simulink model "flightControlSystem"  (R2024b)
settings: Solver=ode3  StartTime=0  StopTime=TFinal  FixedStep=Ts  RelTol=1e-3  EnableMultiTasking=on
model workspace (MAT data in the model file):
  CIRCLE_PTS = [19 19 19]
  ZEROS = [0 0 0 0 0 0 0 0 0 0 0 0 ... (1444 elements, 38x38)]
undefined symbols (not defined in the file or in its folder): codertarget, Controller, DiscIntNeverNeededParam, Discrete, Estimator, g, gray, init, Sensors, Time, Ts, var_acc_angle_N, var_bias_gyr_N, var_gyro_p_N, Vehicle
libraries: simulink x37, slpidlib x4, ctrlSharedLib x4, sharedtransform x3, visiontextngfix x1, parrotlib x1
(part 3 of 3)

== matlab function flightControlSystem/Image Processing System/check_previous_target ==
  data: bw_image input; is_scan output; in_red output; prev_xy input; DISTANCE input; target output; compare output
function [is_scan, in_red, target,compare]  = fcn(bw_image, prev_xy, DISTANCE)

prev_x = prev_xy(1);
prev_y = prev_xy(2);

in_red = bw_image(60, 80);
compare = ~in_red;

is_scan = 0;
target_x = 1;
target_y = 1;
speed = 0;

if prev_x == 0 || prev_y == 0 %scan when prev_coordinates unvalid
    is_scan = 1;
else 
    if bw_image(prev_x, prev_y) == 1 %prev_coordinates in red

        %continue upload new coordinats
        [ref_x, ref_y] = middle_point_of_endless_line(bw_image, prev_x, prev_y);

        target_x = prev_x + ref_x;
        target_y = prev_y + ref_y;
        
        %boundary limit. make path in image
        if target_y > 160
            if target_x == 120 
                target_x = 120 - mod(target_y, 160);
            elseif target_x == 1 
                target_x = mod(target_y, 160);
            end
            target_y = 160;
            
        elseif target_y < 1
            if target_x == 120 
                target_x = 120 - abs(target_y);
            elseif target_x == 1 
                target_x = abs(target_y); 
            end
            target_y = 1;
            
        elseif target_x < 1
            if target_y == 160
                target_y = 160 - abs(target_x);
            elseif target_y == 1
                target_y = abs(target_x);
            end
            target_x = 1;
            
        elseif target_x > 120
            if target_y == 160
                target_y = 160 - (target_x - 120);
            elseif target_y == 1
                target_y = target_x - 120;
            end
            target_x = 120;
        end

        %{
        if target_x < 1   target_x = 1;   end
        if target_x > 120 target_x = 120; end
        if target_y < 1   target_y = 1;   end
        if target_y > 160 target_y = 160; end
        %}
        speed = 100;

    else %target not in red
        
        % endless dissappeared ----------------------------
        if in_red
            distance = line_drawer(60, 80, prev_x, prev_y, bw_image, compare);
            if distance < DISTANCE
                is_scan = 1;
                speed = 0;
            else
                speed = distance;
            end
            
            target_x = prev_x;
            target_y = prev_y;
        else
            is_scan = 1;
            target_x = prev_x;
            target_y = prev_y;
            speed = 40;
        end

    end
end
target = [target_x, target_y, speed];

end % func end



function [ref_x, ref_y] = middle_point_of_endless_line(bw_image, target_x, target_y)

w = edge_number(target_x, target_y);

if w == 1 || w == 3

    % to right
    iter_y = target_y;
    iter_x = target_x;
    plus_or_minus = 1;
    x_or_y = 0; % 0:y   1:x
    distance = 0;

    while bw_image(iter_x, iter_y) == 1
        if x_or_y == 0
            iter_y = iter_y + plus_or_minus;
        else
            iter_x = iter_x + plus_or_minus;
        end
        distance = distance + 1;
        
        if iter_y > 160
            iter_y = 160;
            x_or_y = 1;
            if iter_x == 120
                plus_or_minus = -1;
            elseif iter_x == 1
                plus_or_minus = 1;
            end
        end
        if iter_x < 1
            break;
        elseif iter_x > 120
            break;
        end
    end
    right = distance;

    % to left
    iter_y = target_y;
    iter_x = target_x;
    plus_or_minus = -1;
    x_or_y = 0; % 0:y   1:x
    distance = 0;
    
    while bw_image(iter_x, iter_y) == 1
        if x_or_y == 0
            iter_y = iter_y + plus_or_minus;
        else
            iter_x = iter_x + plus_or_minus;
        end
        distance = distance + 1;

        if iter_y < 1
            iter_y = 1;
            x_or_y = 1;
            if iter_x == 120
                plus_or_minus = -1;
            elseif iter_x == 1
                plus_or_minus = 1;
            end
        end
        if iter_x < 1
            break
        elseif iter_x > 120
            break
        end
    end
    left = distance;
    
    
    ref_x = 0;
    diff = right - left;
    
    if abs(diff) >= 7 && abs(diff) < 25
        ref_y = round(diff/2);
    else
        ref_y = 0;
    end

else % ------------------------- 2 & 4 --------------------------
    % to up
    iter_x = target_x;
    iter_y = target_y;
    plus_or_minus = -1;
    x_or_y = 1; % 0:y   1:x
    distance = 0;
    while bw_image(iter_x, iter_y) == 1
        if x_or_y == 0
            iter_y = iter_y + plus_or_minus;
        else
            iter_x = iter_x + plus_or_minus;
        end
        distance = distance + 1;

        if iter_x < 1
            iter_x = 1;
            x_or_y = 0;
            if iter_y == 1
                plus_or_minus = 1;
            elseif iter_y == 160
                plus_or_minus = -1;
            end
        end
        if iter_y > 160
            break
        elseif iter_y < 1
            break
        end
    end
    up = distance;

    % to down
    iter_x = target_x;
    iter_y = target_y;
    plus_or_minus = 1;
    x_or_y = 1; % 0:y   1:x
    distance = 0;
    while bw_image(iter_x, iter_y) == 1
        if x_or_y == 0
            iter_y = iter_y + plus_or_minus;
        else
            iter_x = iter_x + plus_or_minus;
        end
        distance = distance + 1;
        if iter_x > 120
            x_or_y = 0;
            iter_x = 120;
            if iter_y == 1
                plus_or_minus = 1;
            elseif iter_y == 160
                plus_or_minus = -1;
            end
        end
        if iter_y > 160
            break;
        elseif iter_y < 1
            break;
        end
    end
    down = distance;

    diff = down - up;

    ref_y = 0;
    if abs(diff) >= 7 && abs(diff) < 25
        ref_x = round(diff/2);
    else
        ref_x = 0;
    end
end

end

== matlab function flightControlSystem/Image Processing System/circle_detection_landing ==
  data: bw_image input; detected output; way output; shape input
function [detected, way] = fcn(bw_image, shape)

persistent landing;
if isempty(landing)
    landing = 0;
end

detected = 0;
way = [0 0 0];
land = 0;

%landing order
if landing == 1
    way = [0 0 1];
    detected = 1;

else
    [total_pixel, cord_x, cord_y] = detect_circle(bw_image, shape);
    
    if total_pixel >= 1350%circle detection parameters
        detected = 1;
        center_x = cord_x + 19;%shape parameters
        center_y = cord_y + 19;%shape parameters
    
        %Image boundary limit
        if center_x > 120
            center_x = 120;
        end
        if center_y > 160
            center_y = 160;
        end
        
        %landing order limit
        dif_x = round(60 - center_x);
        dif_y = round(center_y - 80);
        %calculate 
        dist = sqrt(dif_x * dif_x + dif_y * dif_y);
    
        fprintf(' #### CIRCLE - centers: %3.1f %3.1f | dist: %3.1f\n', ...
            center_x, center_y, dist);
    
        if dist < 15
            land = 1;
            landing = 1;
        end
        way_x = dif_x / 130000;
        way_y = dif_y / 130000;
        way = [way_x way_y land];
    end

end

end

function [total_pixel, cord_x, cord_y] = detect_circle(bw_image, shape)

%  total_pixel: sum of number of pixel
%       cord_x: row coordinate of bw_image
%       cord_y: column coordinate of bw_image

[circle_size_x, circle_size_y] = size(shape);
R = 120;  C = 160;

total_pixel = 0;
cord_x = 0;
cord_y = 0;

%circle detection, a slide window
for i = 1:(R - circle_size_x)
    for j = 1:(C - circle_size_y)
        section = bw_image(i:i+circle_size_x-1, j:j+circle_size_y-1);
        result = sum(~xor(section, shape), 'all');
        if result > total_pixel
            total_pixel = result;
            cord_x = i;
            cord_y = j;
        end
    end

end
end

== matlab function flightControlSystem/Image Processing System/visualize_helper ==
  data: r input; R output; g input; b input; way_x input; way_y input; G output; B output; lx input; ly input; rx input; ry input
function [R,G,B] = fcn(r,g,b, way_x, way_y,  lx,ly, rx,ry)

% completely unnecessary block for algorithm, just for visualize

r(60,80) = 255; g(60,80) = 255; b(60,80) = 255;

if way_x >= 1 && way_y >= 1 && way_x <= 120 && way_y <= 160


% -----------------------------------------------
    x1 = 60; y1 = 80;  x2 = way_x;   y2 = way_y;
    swapepd = 0;
    if abs(y2 - y1) > abs(x2 - x1)
        %disp('[swapped] dy bigger')
        swapepd = 1;
        [x1,y1] = deal(y1,x1);
        [x2,y2] = deal(y2,x2);
        xk = 1; yk = 1;
        if (x2 < x1) xk = -1; end
        if (y2 < y1) yk = -1; end
    else
        xk = -1; yk = -1;
        if (x2 > x1) xk = 1; end
        if (y2 > y1) yk = 1; end

    end
    dy = abs(y2-y1);
    dx = abs(x2-x1);
    % --------------------------------------
    m = 2 * dy;
    slope_error = m - 2*dx;
  
    y = y1;
    for x = x1:xk:x2
        if swapepd == 1
            r(y,x) = 255; g(y,x) = 255; b(y,x) = 255;
        else
            r(x,y) = 255; g(x,y) = 255; b(x,y) = 255;
        end
        
   
        slope_error = slope_error + m;
        if (slope_error > 0)
            y = y + yk;
            slope_error = slope_error - 2 * dx;
        end
    end
end




% --------------------------------------------
x1 = 60; y1 = 80; x2 = lx; y2 = ly;
    swapepd = 0;
    if abs(y2 - y1) > abs(x2 - x1)
        %disp('[swapped] dy bigger')
        swapepd = 1;
        [x1,y1] = deal(y1,x1);
        [x2,y2] = deal(y2,x2);
        xk = 1; yk = 1;
        if (x2 < x1) xk = -1; end
        if (y2 < y1) yk = -1; end
    else
        xk = -1; yk = -1;
        if (x2 > x1) xk = 1; end
        if (y2 > y1) yk = 1; end

    end
    dy = abs(y2-y1);
    dx = abs(x2-x1);
    % --------------------------------------
    m = 2 * dy;
    slope_error = m - 2*dx;
  
    y = y1;
    for x = x1:xk:x2
        if swapepd == 1
            g(y,x) = 255;
        else
            g(x,y) = 255;
        end
        
   
        slope_error = slope_error + m;
        if (slope_error > 0)
            y = y + yk;
            slope_error = slope_error - 2 * dx;
        end
    end
% -----------------------------------------

    x1 = 60; y1 = 80; x2 = rx; y2 = ry;
    swapepd = 0;
    if abs(y2 - y1) >= abs(x2 - x1)
        %disp('[swapped] dy bigger')
        swapepd = 1;
        [x1,y1] = deal(y1,x1);
        [x2,y2] = deal(y2,x2);
        xk = 1; yk = 1;
        if (x2 < x1) xk = -1; end
        if (y2 < y1) yk = -1; end
    else
        xk = -1; yk = -1;
        if (x2 > x1) xk = 1; end
        if (y2 > y1) yk = 1; end

    end
    dy = abs(y2-y1);
    dx = abs(x2-x1);
    % --------------------------------------
    m = 2 * dy;
    slope_error = m - 2*dx;
  
    y = y1;
    for x = x1:xk:x2
        if swapepd == 1
            if x <1 break; end
            g(y,x) = 255;
        else
            g(x,y) = 255;
        end
        
   
        slope_error = slope_error + m;
        if (slope_error > 0)
            y = y + yk;
            slope_error = slope_error - 2 * dx;
        end
    end

b(40:80, 60:90) = 200;
R = r;
G = g;
B = b;
end

== matlab function flightControlSystem/Image Processing System/write_or_not ==
  data: target input; way_out output; in_red input; prev_xy input; target_x output; target_y output
function [way_out, target_x, target_y] = fcn(target, in_red, prev_xy)

x = target(1);
y = target(2);
speed = target(3);

if in_red
    X = x;   Y = y;
    target_x = x;  target_y = y;%output as a valid target
else
    X = x;  Y = y; 
    target_x = prev_xy(1);  
    target_y = prev_xy(2);%dont move and start a new loop
end

way_out = [X Y speed];

%fprintf('X = %f | Y = %f\n', target_x, target_y);
end

== matlab function flightControlSystem/Image Processing System/MATLAB Function ==
  data: rgb_image input; bw_image output
function bw_image = red_detection_binarize(rgb_image)
    %  RGB To HSV
    hsv_image = rgb2hsv(rgb_image);

    % HSV Parameters_red
    h_min = 0;    % Min Hue 
    h_max = 0.1;  % Max Hue
    s_min = 0.3;  % Min Saturation
    s_max = 1;    % Max Saturation
    v_min = 0.1;  % Min Value
    v_max = 1;    % Max Value

    % Mask 
    mask1 = (hsv_image(:,:,1) >= h_min & hsv_image(:,:,1) <= h_max) & ...
            (hsv_image(:,:,2) >= s_min & hsv_image(:,:,2) <= s_max) & ...
            (hsv_image(:,:,3) >= v_min & hsv_image(:,:,3) <= v_max);
    mask2 = (hsv_image(:,:,1) >= 0.9 & hsv_image(:,:,1) <= 1) & ...
            (hsv_image(:,:,2) >= s_min & hsv_image(:,:,2) <= s_max) & ...
            (hsv_image(:,:,3) >= v_min & hsv_image(:,:,3) <= v_max);

    % Mask Sum
    red_mask = mask1 | mask2;

    % Keep red  mask, set others black
    masked_rgb = rgb_image;
    masked_rgb(repmat(~red_mask, [1, 1, 3])) = 0;

    % Mask To Grey
    gray_image = rgb2gray(masked_rgb);

    % Grey To Binizaration
    level = graythresh(gray_image);       % Calculate threshold
    bw_image = imbinarize(gray_image, level); 

    % Noise Filter
    %u = bwareaopen(u, 50);
end

== matlab function flightControlSystem/Control System/Controller/Position Controller/Position error transformation (Earth to Body frame) ==
  data: yaw input; xy_err_earth input; xy_err_body output
function xy_err_body = fcn(yaw,xy_err_earth)

transformation = [cos(yaw), sin(yaw); -sin(yaw),  cos(yaw)];
xy_err_body = transformation * xy_err_earth;


end

== matlab function flightControlSystem/Image Processing System/speed_calculator ==
  data: target input; X output; Y output
function [X,Y] = fcn(target)

x = target(1);
y = target(2);
speed = target(3);

if speed == 100
    speed = 200;
elseif speed < 60
    speed = 60;
end


X = (60-x) / 10000000 * speed;
Y = (y-80) / 10000000 * speed;


%fprintf(' --- speed: %f | ', speed); fprintf('vectors: X=%.5f | Y=%.5f\n', X, Y);

end

== matlab function flightControlSystem/Image Processing System/Feedback Control ==
  data: target_x output; prev_xy input; target_y output
function [target_x, target_y] = fcn(prev_xy)

    x = prev_xy(1);
    y = prev_xy(2);
    
    if x == 0 || y == 0 %initial satate
        target_x = 0;
        target_y = 0;
    else
        target_x = 60 + (60 - x) + 1; %1--120
        target_y = 80 + (80 - y) + 1; %2--159
    end

    %fprintf('opposite: %.0f %.0f -> %.0f %.0f\n', x, y, way_x, way_y);
end

== matlab function flightControlSystem/Image Processing System/Position Corrector/center_vector_x ==
  data: bw_image input; slide_x output
function slide_x = fcn(bw_image) 
%input:bw_image,bw_image
%output:slide_x,x direction velocity

%initialize centerpoint
c1 = 60; 
c2 = 80;
left_p = 0;
right_p = 0;
center = bw_image(c1, c2);
compare = ~center;

%find left bound
for i = c2:-1:60 % <---  look left
    if bw_image(c1, i) == compare
        left_p = i;
        break
    end
end

%find right bound
for i = c2:100 % --->   look right
    if bw_image(c1, i) == compare
        right_p = i;
        break
    end
end

slide_x = 0;
if left_p ~= 0 && right_p ~= 0 % in line
    if center == 1
        vr = right_p - c2;  % length right 
        vl = c2 - left_p;   % length left
        diff = vr-vl;%calculate diff to center
        slide_x = get_speed(diff) * 20;%back to center
    end
end
end

function T = get_speed(t)

if t > 0 %too left
    if t < 1 %slowly adjust position when diif is small
        T = 0.000001;
    elseif t < 5
        T = 0.000002;
    elseif t < 10
        T = 0.000003;
    elseif t < 15
        T = 0.000004;
    elseif t < 20
        T = 0.000005;
    else
        T = 0.000006;
    end
else %too right
    if t < -20
        T = -0.000006;
    elseif t < -15
        T = -0.000005;
    elseif t < -10
        T = -0.000004;
    elseif t < -5
        T = -0.000003;
    elseif t < -1
        T = -0.000002;
    else
        T = -0.000001;
    end
end

end

== matlab function flightControlSystem/Image Processing System/range_points ==
  data: x input; x1 output; y input; ref input; y1 output; x2 output; y2 output
function [x1,y1, x2,y2] = get_range_points(x,y, ref)

% x1, y1 are left
% x2, y2 are right 
% according to center-to-edge vector.

W = edge_number(x,y);

if W == 1%up bound
    y1 = y - ref;%To left
    if y1 < 1
        x1 = x - y1;%become left
        y1 = 1;
    else
        x1 = x;
    end

    y2 = y + ref;%To right
    if y2 > 160
        x2 = y2-160;%become right
        y2 = 160;
    else
        x2 = x;
    end
elseif W == 2%left bound
    x1 = x + ref;
    if x1 > 120
        y1 = x1 - 120;
        x1 = 120;
    else
        y1 = y;
    end

    x2 = x - ref;
    if x2 < 1
        y2 = abs(x2) + 1;
        x2 = 1;
    else
        y2 = y;
    end
elseif W == 4%right bound
    x1 = x - ref;
    if x1 < 1
        y1 = 160 + x1;
        x1 = 1;
    else
        y1 = 160;
    end

    x2 = x + ref;
    if x2 > 120
        y2 = 160 - (x2 - 120);
        x2 = 120;
    else
        y2 = y;
    end
elseif W == 3%down bound
    y1 = y + ref;%159+70=229
    if y1 > 160
        x1 = 120 - (y1-160);%51
        y1 = 160;
    else
        x1 = x;
    end

    y2 = y - ref;%89
    if y2 < 1
        x2 = 120 + y2;
        y2 = 1;
    else
        x2 = x;%120
    end
else %initial state and rescan
    x1 = 1; y1 = 1;
    x2 = 1; y2 = 2;
end

%fprintf('range_points: %.0f-%.0f  to  %.0f-%.0f\n', x1,y1, x2,y2);

end

== stateflow chart flightControlSystem/Control System/Path Planning/Chart ==
  state hover
    xout = 0;
    yout = 0;
    zout = -0.5;
  state go
    xout = xout + xin;
    yout = yout + yin;
    zout = -0.5;
  state land
    zout = zout + 0.004;
    xout = xout;
    yout = yout;
  (default) -> hover
  go -> land : [land == 1]
  hover -> go : [after(2, sec)]
  data: xout output; yout output; zout output; yin input; xin input; land input

== matlab function flightControlSystem/Control System/Path Planning/way_parser ==
  data: x output; u input; y output; land output
function [x, y, land] = fcn(u)

x = u(1);
y = u(2);
land = u(3);

end

== matlab function flightControlSystem/Image Processing System/Position Corrector/center_vector_y ==
  data: bw_image input; slide_y output
function slide_y = fcn(bw_image)
c1 = 60; 
c2 = 80;
up_p = 0;
down_p = 0;
center = bw_image(c1,c2);
compare = ~center;
for i = c1:-1:40 % look up
    if bw_image(i, c2) == compare
        up_p = i;
        break
    end
end
for i = c1:80 % look down
    if bw_image(i, c2) == compare
        down_p = i;
        break
    end
end
slide_y = 0;
if up_p ~= 0 && down_p ~= 0  % in line
    if center == 1
        vu = down_p - c1;  %length up
        vd = c1 - up_p;    %length down
        diff = vd-vu;
        
        slide_y = get_speed(diff) * 20;
    end
end

end
function T = get_speed(t)

if t > 0
    if t <= 1
        T = 0.000001;
    elseif t < 5
        T = 0.000002;
    elseif t < 10
        T = 0.000003;
    elseif t < 15
        T = 0.000005;
    elseif t < 20
        T = 0.000005;
    else
        T = 0.000005;
    end
else
    if t < -20
        T = -0.000005;
    elseif t < -15
        T = -0.000005;
    elseif t < -10
        T = -0.000004;
    elseif t <= -5
        T = -0.000003;
    elseif t < -1
        T = -0.000002;
    else
        T = -0.000001;
    end
end
end
